simulink model "sm_parts_box_fillet_tubes"  (R2018b)
settings: Solver=VariableStepAuto  StartTime=0.0  StopTime=10.0  RelTol=1e-3  EnableMultiTasking=on
libraries: Multibody_Parts_Lib x3, sm_lib x2, nesl_utility x1
Description:
  | Copyright 2017-2018 The MathWorks, Inc.
settings Model: Creator=smiller  LastModifiedBy=smiller
settings DataIOCC: LimitDataPoints=on
settings OptimizationCC: LifeSpan=inf
settings DebuggingCC: AllowSymbolicDim=off  LibraryContextMissingDiagnostic=none  SFUnexpectedBacktrackingDiag=warning  SFNoUnconditionalDefaultTransitionDiag=warning  SFExecutionAtInitializationDiag=none
settings SFSimCC: SimUseLocalCustomCode=off
settings RTWCC: RTWUseLocalCustomCode=off
settings CodeAppCC: StateflowObjectComments=on
settings GRTTargetCC: TargetLangStandard=C89/C90 (ANSI)  GeneratePreprocessorConditionals=Disable all
settings ConfigComp: CovMetricSettings=dw  CovHtmlReporting=on  CovSaveCumulativeToWorkspaceVar=on  CovSaveSingleToWorkspaceVar=on  CovExternalEMLEnable=off  CovSFcnEnable=off
settings SimscapeCC: SimscapeNormalizeSystem=off  SimscapeLogType=all  SimscapeLogDataHistory=10000
settings ConfigurationSet: Description=SimMechanics 2G
settings ExplorerConfigSet: InternalSimMechanicsExplorerSettings="<ExplorerConfiguration><canonicalview>planar_xy</canonicalview><AnimationSetting><BasePlaybackSpeed>1.0</BasePlaybackSpeed><PlaybackSpeedFactor>1.0</PlaybackSpeedFactor></AnimationSetting><TilePanel><TileInfo><Tiles Columns=\"1\" Count=\"1\" Rows=\"1\"><Column Left=\"2\" Weight=\"1\"/><Column Left=\"429\"/><Row Top=\"2\" Weight=\"1\"/><Row Top=\"205\"/><Tile Height=\"1\" Width=\"1\" X=\"0\" Y=\"0\"/></Tiles></TileInfo><SceneInfo><SceneViewer><BGColor><R>1</R><G>1</G><B>1</B></BGColor><Camera><DoPerspective>off</DoPerspective><Position><X>-0.65091338015492539</X><Y>0.12983928454150478</Y><Z>0.37574457160893038</Z></Position><Center><X>0.32853998606351043</X><Y>0.02491530511549428</Y><Z>0.20351779684732507</Z></Center><Up><X>0.09727721728061943</X><Y>0.99388336168316949</Y><Z>-0.052278163390663025</Z></Up><ViewLimDist>1</ViewLimDist><YLim>0.15994663632657541</YLim><XLim>0.34462728857994079</XLim></Camera></SceneViewer></SceneInfo></TilePanel><MechEditorPanel><Cameras/><GfxPanelCameraMap/><VideoCreator><PlaybackSpeedRatio>1.0</PlaybackSpeedRatio><FrameRate>30</FrameRate><VideoFormat>Motion JPEG AVI</VideoFormat><FrameSize>auto</FrameSize></VideoCreator></MechEditorPanel></ExplorerConfiguration>"

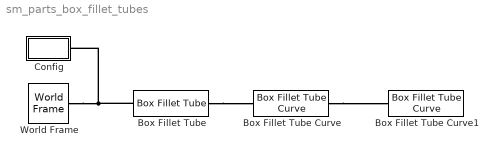
== system sm_parts_box_fillet_tubes ==
  Box Fillet Tube : Multibody_Parts_Lib/Extrusions/Box Fillet Tube  box_ox=0.2  box_ix=0.1  box_oy=0.28  box_iy=0.18  rad_o=0.05  rad_i=0.02  box_len=0.5  box_rho=7000  box_color=[0 0.4 0.6]  box_opc=1
      settings: SourceProductName=Simscape Multibody Parts Library
  Box Fillet Tube Curve : Multibody_Parts_Lib/Extrusions/Box Fillet Tube Curve  box_ox=0.2  box_ix=0.1  box_oy=0.28  box_iy=0.18  rad_o=0.05  rad_i=0.02  arc_rad=0.5  arc_angle=-135  popup_arcdir=Y  box_rho=7000  box_color=[0.8 0.8 0.8]  box_opc=1
      settings: SourceProductName=Simscape Multibody Parts Library
  Box Fillet Tube Curve1 : Multibody_Parts_Lib/Extrusions/Box Fillet Tube Curve  box_ox=0.2  box_ix=0.1  box_oy=0.28  box_iy=0.18  rad_o=0.05  rad_i=0.02  arc_rad=17e-2  arc_angle=60  popup_arcdir=Z  box_rho=7000  box_color=[0 0.4 0.6]  box_opc=1
      settings: SourceProductName=Simscape Multibody Parts Library
  Config : Subsystem
  World Frame : sm_lib/Frames and Transforms/World Frame
  connections:
  World Frame/RConn1 -- Box Fillet Tube/LConn1 -- Config/LConn1
  Box Fillet Tube/RConn1 -- Box Fillet Tube Curve/LConn1
  Box Fillet Tube Curve/RConn1 -- Box Fillet Tube Curve1/LConn1

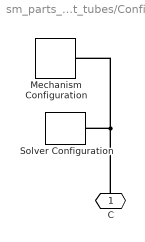
== system sm_parts_box_fillet_tubes/Config ==
  Mechanism Configuration : sm_lib/Utilities/Mechanism Configuration  UniformGravity=Constant  GravityVector=[0 0 -9.80665]  GravityUnits=m/s^2  LinearizationDelta=0.001
  Solver Configuration : nesl_utility/Solver Configuration  PhysicalDomain=network_engine_domain  SubClassName=solver  LeftPortType=input  RightPortType=generic  Tones=[]  Harmonics=[]  SimulateNoise=off  Profile=off  UseLocalSampling=off  EnableSwitchedLinearOptims=on  FrequencyDomain=off  UseCCode=off  RelTol=0.001  AbsTol=1e-06  MinStep=1e-09  ToWorkspace=off  RevertToSquareIcSolve=off  NumHomotopyIterations=100  PhasorMode=off  PhasorModeNumHarmonics=1  DoDC=off  ResidualTolerance=1e-09  UseLocalSolver=off  LocalSolverChoice=NE_BACKWARD_EULER_ADVANCER  LocalSolverSampleTime=0.001  DoFixedCost=off  MaxNonlinIter=3  MaxModeIter=2  LinearAlgebra=Sparse  EquationFormulation=NE_TIME_EF  DelaysMemoryBudget=1024  AutomaticFiltering=on  FilteringTimeConstant=0.001  PartitionStorageMethod=AS_NEEDED  PartitionMemoryBudget=1024
  C : PMIOPort  Side=Left
  connections:
  Mechanism Configuration/RConn1 -- C/RConn1 -- Solver Configuration/RConn1
